simulink model "Example_8_10"  (R2014a)
settings: Solver=FixedStepDiscrete  SolverMode=SingleTasking  StartTime=0.0  StopTime=10  RelTol=1e-3
libraries: dspsrcs4 x1, dsparch4 x1
settings Model: Creator=Lee Edwards  LastModifiedBy=Lee
settings DataIOCC: SignalLoggingSaveFormat=ModelDataLogs  SaveOutput=off  SignalLogging=off  SaveTime=off
settings OptimizationCC: ExpressionDepthLimit=2147483647
settings DebuggingCC: AlgebraicLoopMsg=error  UnderspecifiedInitializationDetection=Classic  SingleTaskRateTransMsg=error  FcnCallInpInsideContextMsg=UseLocalSettings  StateNameClashWarn=warning
settings GRTTargetCC: CombineOutputUpdateFcns=off  GRTInterface=on

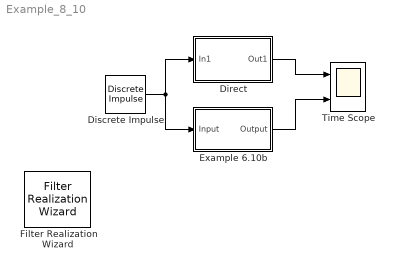
== system Example_8_10 ==
  Direct : Subsystem
  Discrete Impulse : dspsrcs4/Discrete  Impulse  Delay=0  SampleTime=1  FrameSample=1  dataType=double  isSigned=on  wordLen=16  udDataType=sfix(16)  fracBitsMode=Best precision  numFracBits=15  OutDataTypeStr=double  LastOutDataTypeStr=double
  Example 6.10b : Subsystem  Tag=FilterWizardSubSystem
      settings: ErrorFcn=dspFilterRealizedInBasicElemsAlgLoopErrFcnCallback
  Filter Realization Wizard : dsparch4/Filter Realization Wizard
  Time Scope : Scope  NumInputPorts=2
      settings: YMin=-5~-5  YMax=5~5  DataFormat=Structure
  wires:
  Direct/1(Out1) -> Time Scope/1
  Example 6.10b/1(Output) -> Time Scope/2
  Discrete Impulse/1 -> Direct/1(In1), Example 6.10b/1(Input)

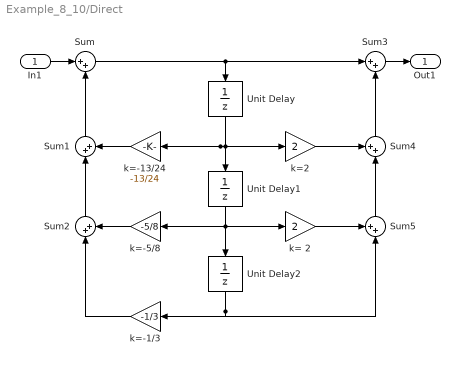
== system Example_8_10/Direct ==
  In1 : Inport
  Sum{,1..3} (4 alike) : Sum  Inputs=|++
  Sum4 : Sum  Inputs=++|
  Sum5 : Sum  Inputs=++|
  Unit Delay : UnitDelay  SampleTime=-1
  Unit Delay1 : UnitDelay  SampleTime=-1
  Unit Delay2 : UnitDelay  SampleTime=-1
  k= 2 : Gain  Gain=2
  k=-1/3 : Gain  Gain=-1/3
  k=-13/24 : Gain  Gain=-13/24
  k=-5/8 : Gain  Gain=-5/8
  k=2 : Gain  Gain=2
  Out1 : Outport
  wires:
  Sum4/1 -> Sum3/2
  k=2/1 -> Sum4/1
  Sum5/1 -> Sum4/2
  k= 2/1 -> Sum5/1
  k=-1/3/1 -> Sum2/1
  Unit Delay2/1 -> k=-1/3/1, Sum5/2
  Sum2/1 -> Sum1/1
  k=-5/8/1 -> Sum2/2
  Sum1/1 -> Sum/2
  k=-13/24/1 -> Sum1/2
  Unit Delay1/1 -> Unit Delay2/1, k=-5/8/1, k= 2/1
  Unit Delay/1 -> Unit Delay1/1, k=-13/24/1, k=2/1
  Sum/1 -> Sum3/1, Unit Delay/1
  In1/1 -> Sum/1
  Sum3/1 -> Out1/1

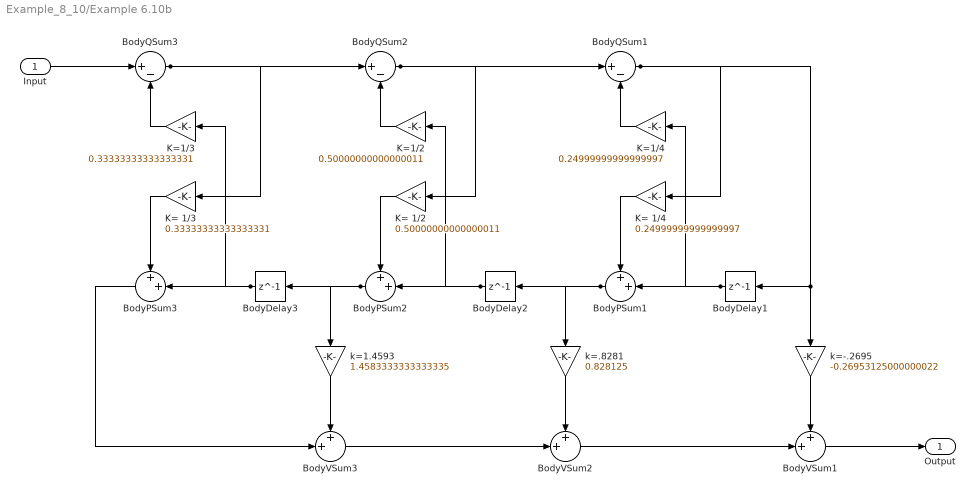
== system Example_8_10/Example 6.10b ==
  Input : Inport
  BodyDelay1 : Delay  DelayLength=1  InputProcessing=Inherited
  BodyDelay2 : Delay  DelayLength=1  InputProcessing=Inherited
  BodyDelay3 : Delay  DelayLength=1  InputProcessing=Inherited
  BodyPSum1 : Sum  Inputs=++|  RndMeth=Nearest  SaturateOnIntegerOverflow=on  OutDataTypeStr=Inherit: Same as first input
  BodyPSum2 : Sum  Inputs=++|  RndMeth=Nearest  SaturateOnIntegerOverflow=on  OutDataTypeStr=Inherit: Same as first input
  BodyPSum3 : Sum  Inputs=++|  RndMeth=Nearest  SaturateOnIntegerOverflow=on  OutDataTypeStr=Inherit: Same as first input
  BodyQSum1 : Sum  Inputs=|+-  RndMeth=Nearest  SaturateOnIntegerOverflow=on  OutDataTypeStr=Inherit: Same as first input
  BodyQSum2 : Sum  Inputs=|+-  RndMeth=Nearest  SaturateOnIntegerOverflow=on  OutDataTypeStr=Inherit: Same as first input
  BodyQSum3 : Sum  Inputs=|+-  RndMeth=Nearest  SaturateOnIntegerOverflow=on  OutDataTypeStr=Inherit: Same as first input
  BodyVSum1 : Sum  Inputs=++|  RndMeth=Nearest  SaturateOnIntegerOverflow=on  OutDataTypeStr=Inherit: Same as first input
  BodyVSum2 : Sum  Inputs=++|  RndMeth=Nearest  SaturateOnIntegerOverflow=on  OutDataTypeStr=Inherit: Same as first input
  BodyVSum3 : Sum  Inputs=++|  RndMeth=Nearest  SaturateOnIntegerOverflow=on  OutDataTypeStr=Inherit: Same as first input
  K= 1/2 : Gain  Gain=0.50000000000000011  ParamDataTypeStr=float('double')  RndMeth=Nearest  SaturateOnIntegerOverflow=on  OutDataTypeStr=Inherit: Same as input
  K= 1/3 : Gain  Gain=0.33333333333333331  ParamDataTypeStr=float('double')  RndMeth=Nearest  SaturateOnIntegerOverflow=on  OutDataTypeStr=Inherit: Same as input
  K= 1/4 : Gain  Gain=0.24999999999999997  ParamDataTypeStr=float('double')  RndMeth=Nearest  SaturateOnIntegerOverflow=on  OutDataTypeStr=Inherit: Same as input
  K=1/2 : Gain  Gain=0.50000000000000011  ParamDataTypeStr=float('double')  RndMeth=Nearest  SaturateOnIntegerOverflow=on  OutDataTypeStr=Inherit: Same as input
  K=1/3 : Gain  Gain=0.33333333333333331  ParamDataTypeStr=float('double')  RndMeth=Nearest  SaturateOnIntegerOverflow=on  OutDataTypeStr=Inherit: Same as input
  K=1/4 : Gain  Gain=0.24999999999999997  ParamDataTypeStr=float('double')  RndMeth=Nearest  SaturateOnIntegerOverflow=on  OutDataTypeStr=Inherit: Same as input
  k=-.2695 : Gain  Gain=-0.26953125000000022  ParamDataTypeStr=float('double')  RndMeth=Nearest  SaturateOnIntegerOverflow=on  OutDataTypeStr=Inherit: Same as input
  k=.8281 : Gain  Gain=0.828125  ParamDataTypeStr=float('double')  RndMeth=Nearest  SaturateOnIntegerOverflow=on  OutDataTypeStr=Inherit: Same as input
  k=1.4593 : Gain  Gain=1.4583333333333335  ParamDataTypeStr=float('double')  RndMeth=Nearest  SaturateOnIntegerOverflow=on  OutDataTypeStr=Inherit: Same as input
  Output : Outport
  wires:
  BodyQSum1/1 -> K= 1/4/1, BodyDelay1/1, k=-.2695/1
  K=1/4/1 -> BodyQSum1/2
  K= 1/4/1 -> BodyPSum1/1
  BodyPSum1/1 -> BodyDelay2/1, k=.8281/1
  BodyDelay1/1 -> K=1/4/1, BodyPSum1/2
  k=-.2695/1 -> BodyVSum1/1
  BodyVSum1/1 -> Output/1
  BodyQSum2/1 -> K= 1/2/1, BodyQSum1/1
  K=1/2/1 -> BodyQSum2/2
  K= 1/2/1 -> BodyPSum2/1
  BodyPSum2/1 -> BodyDelay3/1, k=1.4593/1
  BodyDelay2/1 -> K=1/2/1, BodyPSum2/2
  k=.8281/1 -> BodyVSum2/1
  BodyVSum2/1 -> BodyVSum1/2
  BodyQSum3/1 -> K= 1/3/1, BodyQSum2/1
  K=1/3/1 -> BodyQSum3/2
  K= 1/3/1 -> BodyPSum3/1
  BodyPSum3/1 -> BodyVSum3/2
  BodyDelay3/1 -> K=1/3/1, BodyPSum3/2
  k=1.4593/1 -> BodyVSum3/1
  BodyVSum3/1 -> BodyVSum2/2
  Input/1 -> BodyQSum3/1
